simulink model "problem3"  (R2020b)
settings: Solver=VariableStepAuto  StartTime=0.0  StopTime=10.0  RelTol=1e-3
undefined symbols (not defined in the file): Cf, Cr, Iyy, Kf, Kr, Lf, Lr, sigbuilder_block
settings Model: Creator=Nitin  LastModifiedBy=Nitin

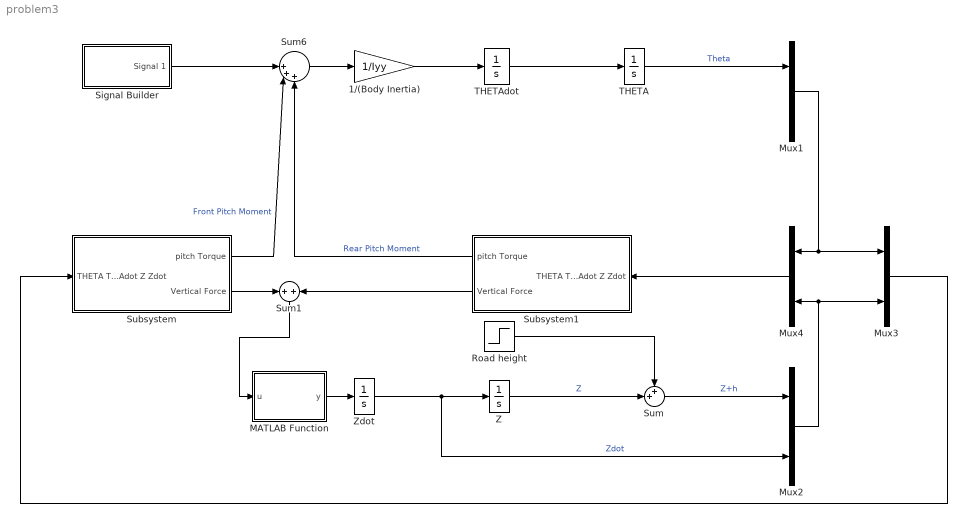
== system problem3 ==
  1/(Body Inertia) : Gain  Gain=1/Iyy  SaturateOnIntegerOverflow=on  OutDataTypeStr=Inherit: Same as input  ParamDataTypeStr=Inherit: Same as input
  MATLAB Function : MATLAB Function  TreatAsAtomicUnit=on
  Mux{1..4} (4 alike) : Mux  Inputs=2
      settings: DisplayOption=signals
  Road height : Step  Time=7  After=0.01  SampleTime=0
  Signal Builder : Subsystem  Tag=STV Subsys  LoadFcn=sigbuilder_block('load');  StartFcn=sigbuilder_block('start');  StopFcn=sigbuilder_block('stop');  ClipboardFcn=sigbuilder_block('clipboard');  mask(Sigbuilder block){tuvar=[0:10]}
      mask help: Simulink:masks:SigbuilderBlock_MD
      mask init:
      | if ~strcmp(get_param(bdroot(gcbh),'SimulationStatus'),'stopped') tuvar = sigbuilder_block('maskInit'); end
      settings: CopyFcn=sigbuilder_block('copy');  DeleteFcn=sigbuilder_block('delete');  ModelCloseFcn=sigbuilder_block('modelClose');  PreSaveFcn=sigbuilder_block('preSave');  PauseFcn=sigbuilder_block('pause');  ContinueFcn=sigbuilder_block('continue');  NameChangeFcn=sigbuilder_block('namechange');  OpenFcn=sigbuilder_block('open',[437.6 199.2 550.4 400 ]);  CloseFcn=sigbuilder_block('close');
      mask Display: plot(0, 0, 100, 100,[2, 2, 32, 32, 2], [68, 8, 8, 68, 68],[32, 2], [38, 38], [32, 19, 2],[53, 60, 44], [32, 17, 17, 2],[16, 16, 31, 31]);txt = getActiveGroup(gcbh);text(2, 100, txt,'verticalAlignment', 'top');
  Subsystem : Subsystem
  Subsystem1 : Subsystem
  Sum : Sum  Inputs=++|
  Sum1 : Sum
  Sum6 : Sum  Inputs=||+++  InputSameDT=on  SaturateOnIntegerOverflow=on  OutDataTypeStr=Inherit: Same as first input
  THETA : Integrator  InitialCondition=-8.7e-20
  THETAdot : Integrator  InitialCondition=8.04e-28
  Z : Integrator  InitialCondition=-0.12
  Zdot : Integrator
  wires:
  Subsystem1/1(pitch Torque) -> Sum6/3  "Rear Pitch Moment"
  Subsystem/1(pitch Torque) -> Sum6/2  "Front Pitch Moment"
  THETA/1 -> Mux1/1  "Theta"
  Sum6/1 -> 1/(Body Inertia)/1
  Z/1 -> Sum/2  "Z"
  Sum/1 -> Mux2/1  "Z+h"
  Zdot/1 -> Mux2/2, Z/1  "Zdot"
  MATLAB Function/1(y) -> Zdot/1
  THETAdot/1 -> THETA/1
  1/(Body Inertia)/1 -> THETAdot/1
  Mux2/1 -> Mux3/2, Mux4/2
  Mux1/1 -> Mux3/1, Mux4/1
  Mux3/1 -> Subsystem/1(THETA THETAdot Z Zdot)
  Mux4/1 -> Subsystem1/1(THETA THETAdot Z Zdot)
  Subsystem/2(Vertical Force) -> Sum1/1
  Subsystem1/2(Vertical Force) -> Sum1/2
  Signal Builder/1(Signal 1) -> Sum6/1
  Sum1/1 -> MATLAB Function/1(u)
  Road height/1 -> Sum/1

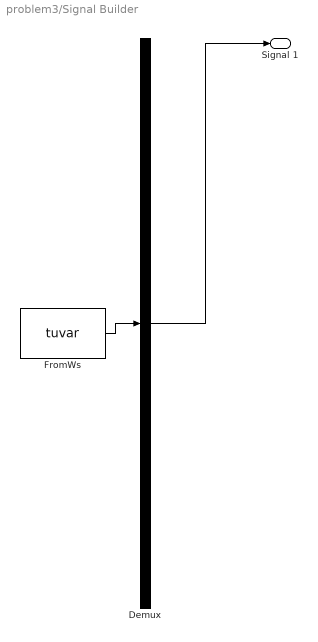
== system problem3/Signal Builder ==
  Demux : Demux  Tag=STV Demux  Outputs=1
      settings: DisplayOption=none
  FromWs : FromWorkspace  Tag=STV FromWs  VariableName=tuvar
      SigBuilderData=|
      | common.afterFinalStr = 'Extrapolate'
      | common.sampleTime = 0
      | dataSet.timeRange = [0 10]
      | dataSet.name = 'Group 1'
      | sbobj.Groups.Name = 'Group 1'
      | sbobj.Groups.Signals.Name = 'Signal 1'
      | sbobj.Groups.Signals.XData = [0 5 5 10]
      | sbobj.Groups.Signals.YData = [0 0 1 1]
  Signal 1 : Outport  Tag=STV Outport
  wires:
  Demux/1 -> Signal 1/1
  FromWs/1 -> Demux/1

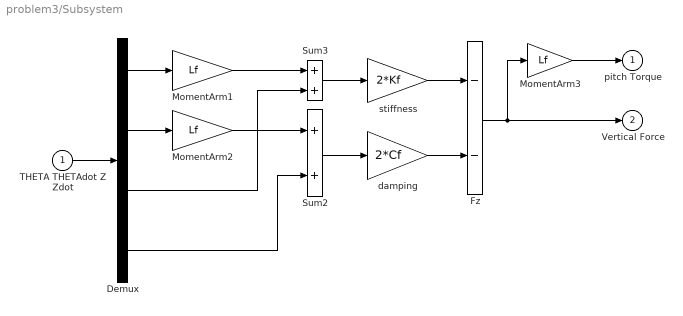
== system problem3/Subsystem ==
  THETA THETAdot Z Zdot : Inport
  Demux : Demux
      settings: DisplayOption=none
  Fz : Sum  Inputs=--  InputSameDT=on  SaturateOnIntegerOverflow=on  OutDataTypeStr=Inherit: Same as first input
  MomentArm1 : Gain  Gain=Lf  SaturateOnIntegerOverflow=on  OutDataTypeStr=Inherit: Same as input  ParamDataTypeStr=Inherit: Same as input
  MomentArm2 : Gain  Gain=Lf  SaturateOnIntegerOverflow=on  OutDataTypeStr=Inherit: Same as input  ParamDataTypeStr=Inherit: Same as input
  MomentArm3 : Gain  Gain=Lf  SaturateOnIntegerOverflow=on  OutDataTypeStr=Inherit: Same as input  ParamDataTypeStr=Inherit: Same as input
  Sum2 : Sum  InputSameDT=on  SaturateOnIntegerOverflow=on  OutDataTypeStr=Inherit: Same as first input
  Sum3 : Sum  InputSameDT=on  SaturateOnIntegerOverflow=on  OutDataTypeStr=Inherit: Same as first input
  damping : Gain  Gain=2*Cf  SaturateOnIntegerOverflow=on  OutDataTypeStr=Inherit: Same as input  ParamDataTypeStr=Inherit: Same as input
  stiffness : Gain  Gain=2*Kf  SaturateOnIntegerOverflow=on  OutDataTypeStr=Inherit: Same as input  ParamDataTypeStr=Inherit: Same as input
  pitch Torque : Outport  VectorParamsAs1DForOutWhenUnconnected=off
  Vertical Force : Outport  Port=2  VectorParamsAs1DForOutWhenUnconnected=off
  wires:
  Demux/2 -> MomentArm2/1
  Demux/3 -> Sum3/2
  Demux/4 -> Sum2/2
  stiffness/1 -> Fz/1
  MomentArm2/1 -> Sum2/1
  MomentArm1/1 -> Sum3/1
  MomentArm3/1 -> pitch Torque/1
  Sum3/1 -> stiffness/1
  damping/1 -> Fz/2
  Fz/1 -> Vertical Force/1, MomentArm3/1
  THETA THETAdot Z Zdot/1 -> Demux/1
  Sum2/1 -> damping/1
  Demux/1 -> MomentArm1/1

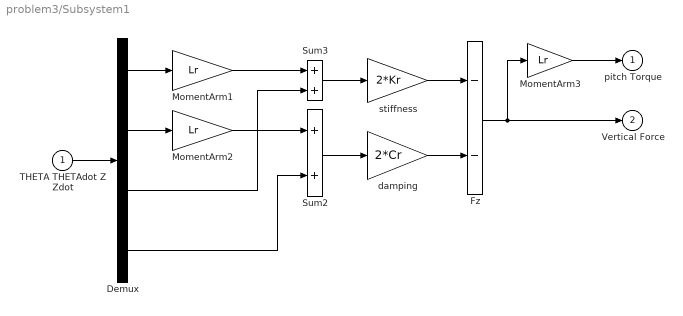
== system problem3/Subsystem1 ==
  THETA THETAdot Z Zdot : Inport
  Demux : Demux
      settings: DisplayOption=none
  Fz : Sum  Inputs=--  InputSameDT=on  SaturateOnIntegerOverflow=on  OutDataTypeStr=Inherit: Same as first input
  MomentArm1 : Gain  Gain=Lr  SaturateOnIntegerOverflow=on  OutDataTypeStr=Inherit: Same as input  ParamDataTypeStr=Inherit: Same as input
  MomentArm2 : Gain  Gain=Lr  SaturateOnIntegerOverflow=on  OutDataTypeStr=Inherit: Same as input  ParamDataTypeStr=Inherit: Same as input
  MomentArm3 : Gain  Gain=Lr  SaturateOnIntegerOverflow=on  OutDataTypeStr=Inherit: Same as input  ParamDataTypeStr=Inherit: Same as input
  Sum2 : Sum  InputSameDT=on  SaturateOnIntegerOverflow=on  OutDataTypeStr=Inherit: Same as first input
  Sum3 : Sum  InputSameDT=on  SaturateOnIntegerOverflow=on  OutDataTypeStr=Inherit: Same as first input
  damping : Gain  Gain=2*Cr  SaturateOnIntegerOverflow=on  OutDataTypeStr=Inherit: Same as input  ParamDataTypeStr=Inherit: Same as input
  stiffness : Gain  Gain=2*Kr  SaturateOnIntegerOverflow=on  OutDataTypeStr=Inherit: Same as input  ParamDataTypeStr=Inherit: Same as input
  pitch Torque : Outport  VectorParamsAs1DForOutWhenUnconnected=off
  Vertical Force : Outport  Port=2  VectorParamsAs1DForOutWhenUnconnected=off
  wires:
  Demux/2 -> MomentArm2/1
  Demux/3 -> Sum3/2
  Demux/4 -> Sum2/2
  stiffness/1 -> Fz/1
  MomentArm2/1 -> Sum2/1
  MomentArm1/1 -> Sum3/1
  MomentArm3/1 -> pitch Torque/1
  Sum3/1 -> stiffness/1
  damping/1 -> Fz/2
  Fz/1 -> Vertical Force/1, MomentArm3/1
  THETA THETAdot Z Zdot/1 -> Demux/1
  Sum2/1 -> damping/1
  Demux/1 -> MomentArm1/1

== matlab function problem3/MATLAB Function ==
  data: u input; y output
function y = fcn(u)

y = [(u*(1/Mb))+(-9.81)];
